simulink model "netra_rakshak_telemedicine"  (R2026a)
settings: Solver=VariableStepAuto
settings Model: Creator=devku  LastModifiedBy=devku

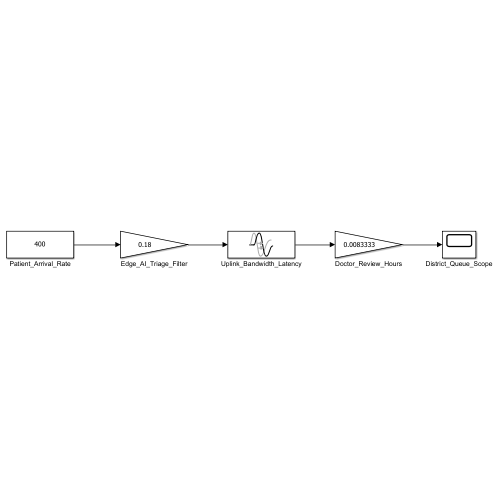
[thumbnail: Simulink's stored preview of the top-level diagram]
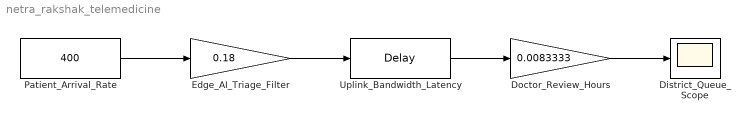
== system netra_rakshak_telemedicine ==
  District_Queue_Scope : Scope
  Doctor_Review_Hours : Gain  Gain=0.0083333
  Edge_AI_Triage_Filter : Gain  Gain=0.18
  Patient_Arrival_Rate : Constant  Value=400
  Uplink_Bandwidth_Latency : TransportDelay  DelayTime=3.6351
  wires:
  Patient_Arrival_Rate/1 -> Edge_AI_Triage_Filter/1
  Edge_AI_Triage_Filter/1 -> Uplink_Bandwidth_Latency/1
  Uplink_Bandwidth_Latency/1 -> Doctor_Review_Hours/1
  Doctor_Review_Hours/1 -> District_Queue_Scope/1
